simulink model "mc_att_control"  (R2021a)
settings: Solver=FixedStepAuto  StartTime=0.0  StopTime=10.0  RelTol=1e-3
undefined symbols (not defined in the file): deg, DiscIntNeverNeededParam, MC_ACRO_EXPO, MC_ACRO_EXPO_Y, MC_ACRO_P_MAX, MC_ACRO_R_MAX, MC_ACRO_SUPEXPO, MC_ACRO_SUPEXPOY, MC_ACRO_Y_MAX, MC_AIRMODE, MC_BAT_SCALE_EN, MC_MAN_TILT_TAU, MC_PITCH_P, MC_PITCHRATE_D, MC_PITCHRATE_FF, MC_PITCHRATE_I, MC_PITCHRATE_K, MC_PITCHRATE_MAX, MC_PITCHRATE_P, MC_PR_INT_LIM, MC_ROLL_P, MC_ROLLRATE_D, MC_ROLLRATE_FF, MC_ROLLRATE_I, MC_ROLLRATE_K, MC_ROLLRATE_MAX, MC_ROLLRATE_P, MC_RR_INT_LIM, MC_YAW_P, MC_YAW_WEIGHT, MC_YAWRATE_D, MC_YAWRATE_FF, MC_YAWRATE_I, MC_YAWRATE_K, MC_YAWRATE_MAX, MC_YAWRATE_P, MC_YR_INT_LIM, MPC_MAN_TILT_MAX, MPC_MAN_Y_MAX, MPC_MANTHR_MIN, MPC_THR_CURVE, MPC_THR_HOVER, MPC_THR_MAX, param_mpc_thr_hover, param_mpc_thr_max, rad, roll_pitch_yaw, s, VEHICLE_TYPE_ROTARY_WING
libraries: simulink x22, aerolibutil x8, sharedtransform x6, aerolibconvert2 x3, vrlib x2, sharedutil x1
(part 2 of 2)

== system mc_att_control/Manual//Stabilized Setpoint/input mapping for roll& pitch setpoint/vector limitation ==
  v : Inport
  Divide : Product  Inputs=*/
  Dot Product2 : DotProduct  InputSameDT=on  OutDataTypeStr=Inherit: Inherit via internal rule
  Gain : Gain  Gain=MPC_MAN_TILT_MAX
      settings: AttributesFormatString=%<Gain>
  Sqrt1 : Sqrt  SaturateOnIntegerOverflow=on
  Switch1 : Switch  Criteria=u2 > Threshold  Threshold=MPC_MAN_TILT_MAX
  v_limited : Outport
  wires:
  v/1 -> Gain/1, Switch1/3, Dot Product2/2, Dot Product2/1
  Switch1/1 -> v_limited/1
  Dot Product2/1 -> Sqrt1/1
  Sqrt1/1 -> Divide/2, Switch1/2  "v_norm"
  Divide/1 -> Switch1/1
  Gain/1 -> Divide/1

== system mc_att_control/Manual//Stabilized Setpoint/vtol modify roll//pitch/Wrap -pi~pi ==
  In1 : Inport
  Constant1 : Constant  Value=2*pi  OutDataTypeStr=single
  Mod : Math  Operator=mod  SaturateOnIntegerOverflow=on
  Sum1 : Sum  Inputs=|+-
  Switch : Switch  Criteria=u2 > Threshold  Threshold=pi
  Out1 : Outport
  wires:
  Sum1/1 -> Switch/1
  Mod/1 -> Switch/3, Sum1/1, Switch/2
  Constant1/1 -> Sum1/2, Mod/2
  Switch/1 -> Out1/1
  In1/1 -> Mod/1

== system mc_att_control/Rate Control/I/mixer saturation ==
  rate_err : Inport
  Bitwise Operator : simulink/Logic and Bit Operations/Bitwise Operator  logicop=AND  UseBitMask=on  BitMask=bin2dec('00001000')  BitMaskRealWorld=Stored Integer
  Bitwise Operator1 : simulink/Logic and Bit Operations/Bitwise Operator  logicop=AND  UseBitMask=on  BitMask=bin2dec('00010000')  BitMaskRealWorld=Stored Integer
  Bitwise Operator2 : simulink/Logic and Bit Operations/Bitwise Operator  logicop=AND  UseBitMask=on  BitMask=bin2dec('00100000')  BitMaskRealWorld=Stored Integer
  Bitwise Operator3 : simulink/Logic and Bit Operations/Bitwise Operator  logicop=AND  UseBitMask=on  BitMask=bin2dec('01000000')  BitMaskRealWorld=Stored Integer
  Bitwise Operator4 : simulink/Logic and Bit Operations/Bitwise Operator  logicop=AND  UseBitMask=on  BitMask=bin2dec('10000000')  BitMaskRealWorld=Stored Integer
  Bitwise Operator5 : simulink/Logic and Bit Operations/Bitwise Operator  logicop=AND  UseBitMask=on  BitMask=bin2dec('100000000')  BitMaskRealWorld=Stored Integer
  Compare To Constant : simulink/Logic and Bit Operations/Compare To Constant  relop=>=  const=0.0  OutDataTypeStr=boolean
  Compare To Constant1 : simulink/Logic and Bit Operations/Compare To Constant  relop=<  const=0.0  OutDataTypeStr=boolean
  Constant : Constant  Value=[0 0 0]  OutDataTypeStr=single
  Logical Operator : Logic  AllPortsSameDT=off  OutDataTypeStr=boolean
  Logical Operator1 : Logic  AllPortsSameDT=off  OutDataTypeStr=boolean
  Logical Operator2 : Logic  Operator=OR  AllPortsSameDT=off  OutDataTypeStr=boolean
  Mux : Mux  Inputs=3
  Mux1 : Mux  Inputs=3
  Switch : Switch  Criteria=u2 ~= 0
  rate_err1 : InportShadow
  rate_err_limited : Outport
  wires:
  [saturation_status] -> Bitwise Operator5/1, Bitwise Operator3/1, Bitwise Operator1/1, Bitwise Operator/1, Bitwise Operator2/1, Bitwise Operator4/1
  Bitwise Operator/1 -> Mux/1  "roll_pos"
  Bitwise Operator1/1 -> Mux1/1  "roll_neg"
  Bitwise Operator2/1 -> Mux/2  "pitch_pos"
  Bitwise Operator3/1 -> Mux1/2  "pitch_neg"
  Bitwise Operator4/1 -> Mux/3  "yaw_pos"
  Bitwise Operator5/1 -> Mux1/3  "yaw_neg"
  Mux/1 -> [pos]
  Mux1/1 -> [neg]
  Compare To Constant/1 -> Logical Operator/2
  rate_err/1 -> Compare To Constant/1, Compare To Constant1/1
  [pos] -> Logical Operator/1
  [neg] -> Logical Operator1/2
  Compare To Constant1/1 -> Logical Operator1/1
  Logical Operator/1 -> Logical Operator2/1
  Logical Operator1/1 -> Logical Operator2/2
  Logical Operator2/1 -> Switch/2
  Constant/1 -> Switch/1
  rate_err1/1 -> Switch/3
  Switch/1 -> rate_err_limited/1

== system mc_att_control/Manual//Stabilized Setpoint/input mapping for roll& pitch setpoint/man_yaw_sp/Wrap -pi~pi ==
  In1 : Inport
  Constant1 : Constant  Value=2*pi  OutDataTypeStr=single
  Mod : Math  Operator=mod  SaturateOnIntegerOverflow=on
  Sum1 : Sum  Inputs=|+-
  Switch : Switch  Criteria=u2 > Threshold  Threshold=pi
  Out1 : Outport
  wires:
  Sum1/1 -> Switch/1
  Mod/1 -> Switch/3, Sum1/1, Switch/2
  Constant1/1 -> Sum1/2, Mod/2
  Switch/1 -> Out1/1
  In1/1 -> Mod/1
